simulink model "kirschFilter"  (R2024a)
settings: Solver=FixedStepDiscrete  StartTime=0.0  StopTime=1  RelTol=1e-3
undefined symbols (not defined in the file): north, northWest, southWest, west
libraries: visionsinks x4, visionsources x1
Description:
  | Sobel Edge Detection Using the MATLAB(R) Function Block
  | This example shows how to use HDL Coder(TM) to check,
  | generate, and verify HDL code for a Sobel Edge Detection
  | block built using the MATLAB Function block.
settings Model: FPTRunName=Active  Creator=The MathWorks, Inc.  LastModifiedBy=dskap
settings SolverCC: AlgebraicLoopSolver=TrustRegion
settings DataIOCC: LimitDataPoints=on  SaveFormat=Array  SignalLogging=off  ReturnWorkspaceOutputs=off
settings OptimizationCC: BlockReduction=off  ConditionallyExecuteInputs=off  DefaultParameterBehavior=Inlined  ExpressionDepthLimit=2147483647  InitFltsAndDblsToZero=on  EfficientMapNaN2IntZero=off  LifeSpan=inf
settings DebuggingCC: AlgebraicLoopMsg=error  SaveWithParameterizedLinksMsg=none  UnderspecifiedInitializationDetection=Classic  MergeDetectMultiDrivingBlocksExec=none  SignalResolutionControl=TryResolveAllWithWarning  MultiTaskDSMMsg=warning  MultiTaskCondExecSysMsg=none  SingleTaskRateTransMsg=error  IntegerOverflowMsg=none  ParameterPrecisionLossMsg=none  FcnCallInpInsideContextMsg=warning  UnconnectedInputMsg=warning  UnconnectedOutputMsg=warning  UnconnectedLineMsg=warning  AllowSymbolicDim=off  StateNameClashWarn=warning  StrictBusMsg=ErrorOnBusTreatedAsVector  SFUnexpectedBacktrackingDiag=warning  SFNoUnconditionalDefaultTransitionDiag=warning  SFExecutionAtInitializationDiag=none  IntegerSaturationMsg=none  ArithmeticOperatorsInVariantConditions=warning
settings HardwareCC: ProdBitPerPointer=32  ProdBitPerSizeT=32  ProdBitPerPtrDiffT=32  ProdLargestAtomicFloat=None  ProdIntDivRoundTo=Undefined  ProdEndianess=Unspecified  ProdWordSize=32  ProdHWDeviceType=ASIC/FPGA  TargetHWDeviceType=32-bit Generic  ProdEqTarget=off
settings ModelReferenceCC: EnableRefExpFcnMdlSchedulingChecks=on  PropagateSignalLabelsOutOfModel=off
settings SFSimCC: SimUseLocalCustomCode=off  CustomCodeUndefinedFunction=UseInterfaceOnly
settings RTWCC: RTWUseLocalCustomCode=off  GPUComputeCapability=3.5  DLArmComputeVersion=19.05
settings CodeAppCC: StateflowObjectComments=on
settings GRTTargetCC: TargetFcnLib=ansi_tfl_tmw.mat  TargetLangStandard=C89/C90 (ANSI)  CombineOutputUpdateFcns=off  GRTInterface=on
settings ConfigComp: CovMetricSettings=dw  CovSaveCumulativeToWorkspaceVar=on  CovSaveSingleToWorkspaceVar=on  CovExternalEMLEnable=off

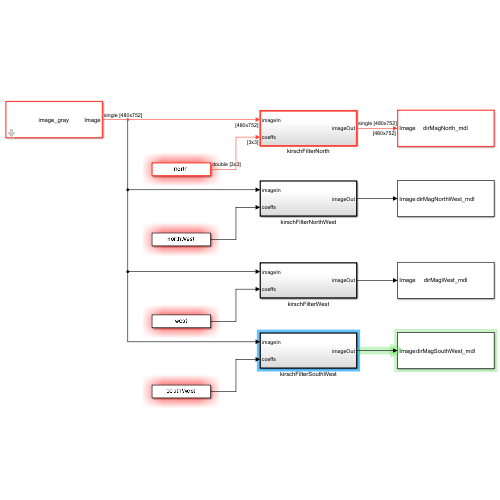
[thumbnail: Simulink's stored preview of the top-level diagram]
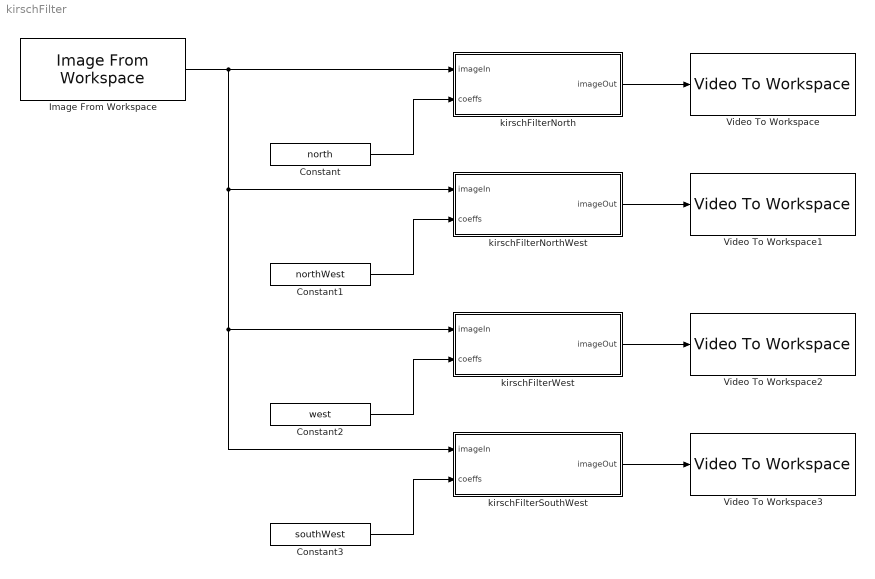
== system kirschFilter ==
  Constant : Constant  Value=north  SampleTime=-1
  Constant1 : Constant  Value=northWest  SampleTime=-1
  Constant2 : Constant  Value=west  SampleTime=-1
  Constant3 : Constant  Value=southWest  SampleTime=-1
  Image From Workspace : visionsources/Image From Workspace  Tag=vipblks_nd  ImageValue=image_gray  Ts=1  imagePorts=One multidimensional signal  OutPortLabels=R|G|B  ImageDataType=Inherit from 'Value'  Signed=on  WordLength=16  sdImageDataType=sfix(16)  FractionLengthMode=User-defined  FractionLength=15
  Video To Workspace : visionsinks/Video To Workspace  VariableName=dirMagNorth_mdl  NumInputs=1  DataLimit=1  DecimationFactor=1  LogFi=off  InPortLabels=R|G|B
  Video To Workspace1 : visionsinks/Video To Workspace  VariableName=dirMagNorthWest_mdl  NumInputs=1  DataLimit=1  DecimationFactor=1  LogFi=off  InPortLabels=R|G|B
  Video To Workspace2 : visionsinks/Video To Workspace  VariableName=dirMagWest_mdl  NumInputs=1  DataLimit=1  DecimationFactor=1  LogFi=off  InPortLabels=R|G|B
  Video To Workspace3 : visionsinks/Video To Workspace  VariableName=dirMagSouthWest_mdl  NumInputs=1  DataLimit=1  DecimationFactor=1  LogFi=off  InPortLabels=R|G|B
  kirschFilterNorth : Subsystem  TreatAsAtomicUnit=on
  kirschFilterNorthWest : Subsystem  TreatAsAtomicUnit=on
  kirschFilterSouthWest : Subsystem  TreatAsAtomicUnit=on
  kirschFilterWest : Subsystem  TreatAsAtomicUnit=on
  wires:
  Image From Workspace/1 -> kirschFilterNorthWest/1(imageIn), kirschFilterWest/1(imageIn), kirschFilterSouthWest/1(imageIn), kirschFilterNorth/1(imageIn)
  kirschFilterNorth/1(imageOut) -> Video To Workspace/1
  Constant/1 -> kirschFilterNorth/2(coeffs)
  kirschFilterNorthWest/1(imageOut) -> Video To Workspace1/1
  Constant1/1 -> kirschFilterNorthWest/2(coeffs)
  kirschFilterSouthWest/1(imageOut) -> Video To Workspace3/1
  Constant3/1 -> kirschFilterSouthWest/2(coeffs)
  kirschFilterWest/1(imageOut) -> Video To Workspace2/1
  Constant2/1 -> kirschFilterWest/2(coeffs)

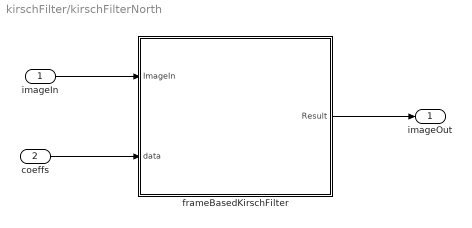
== system kirschFilter/kirschFilterNorth ==
  imageIn : Inport
  coeffs : Inport  Port=2
  frameBasedKirschFilter : MATLAB Function  TreatAsAtomicUnit=on
  imageOut : Outport
  wires:
  imageIn/1 -> frameBasedKirschFilter/1(ImageIn)
  frameBasedKirschFilter/1(Result) -> imageOut/1
  coeffs/1 -> frameBasedKirschFilter/2(data)

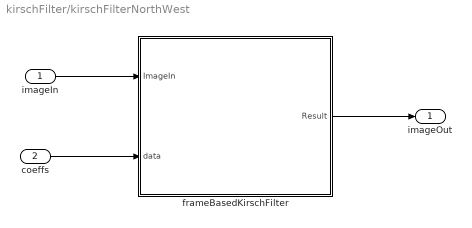
== system kirschFilter/kirschFilterNorthWest ==
  imageIn : Inport
  coeffs : Inport  Port=2
  frameBasedKirschFilter : MATLAB Function  TreatAsAtomicUnit=on
  imageOut : Outport
  wires:
  imageIn/1 -> frameBasedKirschFilter/1(ImageIn)
  frameBasedKirschFilter/1(Result) -> imageOut/1
  coeffs/1 -> frameBasedKirschFilter/2(data)

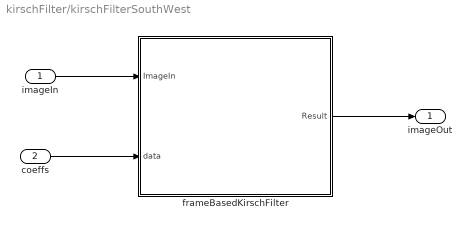
== system kirschFilter/kirschFilterSouthWest ==
  imageIn : Inport
  coeffs : Inport  Port=2
  frameBasedKirschFilter : MATLAB Function  TreatAsAtomicUnit=on
  imageOut : Outport
  wires:
  imageIn/1 -> frameBasedKirschFilter/1(ImageIn)
  frameBasedKirschFilter/1(Result) -> imageOut/1
  coeffs/1 -> frameBasedKirschFilter/2(data)

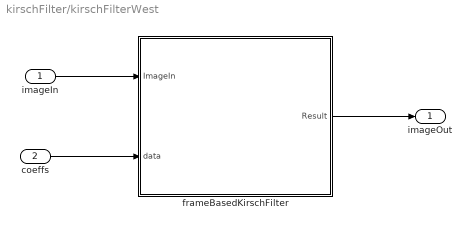
== system kirschFilter/kirschFilterWest ==
  imageIn : Inport
  coeffs : Inport  Port=2
  frameBasedKirschFilter : MATLAB Function  TreatAsAtomicUnit=on
  imageOut : Outport
  wires:
  imageIn/1 -> frameBasedKirschFilter/1(ImageIn)
  frameBasedKirschFilter/1(Result) -> imageOut/1
  coeffs/1 -> frameBasedKirschFilter/2(data)

== matlab function kirschFilter/kirschFilterNorthWest/frameBasedKirschFilter ==
  data: Result output; ImageIn input; data input
function Result   = frameBasedKirschFilter(ImageIn, data)
    Result = hdl.npufun(@kirschKernel, [3 3], ImageIn,'NonSampleInput', data); 
end
 
function e = kirschKernel(in,data)
    temp = in.*data;
    e = abs(sum(sum(temp)));
end

== matlab function kirschFilter/kirschFilterNorth/frameBasedKirschFilter ==
  data: Result output; ImageIn input; data input
function Result   = frameBasedKirschFilter(ImageIn, data)
    Result = hdl.npufun(@kirschKernel, [3 3], ImageIn,'NonSampleInput', data); 
end
 
function e = kirschKernel(in,data)
    temp = in.*data;
    e = abs(sum(sum(temp)));
end

== matlab function kirschFilter/kirschFilterWest/frameBasedKirschFilter ==
  data: Result output; ImageIn input; data input
function Result   = frameBasedKirschFilter(ImageIn, data)
    Result = hdl.npufun(@kirschKernel, [3 3], ImageIn,'NonSampleInput', data); 
end
 
function e = kirschKernel(in,data)
    temp = in.*data;
    e = abs(sum(sum(temp)));
end

== matlab function kirschFilter/kirschFilterSouthWest/frameBasedKirschFilter ==
  data: Result output; ImageIn input; data input
function Result   = frameBasedKirschFilter(ImageIn, data)
    Result = hdl.npufun(@kirschKernel, [3 3], ImageIn,'NonSampleInput', data); 
end
 
function e = kirschKernel(in,data)
    temp = in.*data;
    e = abs(sum(sum(temp)));
end
